simulink model "ansiOct"  (R2018a)
settings: Solver=VariableStepAuto  StartTime=0.0  StopTime=0.1  RelTol=1e-3
undefined symbols (not defined in the file or in its folder): fdesignblkfcn, G1, G2, G3, G4, G5, G6, G7, G8, gcbh, get, T
libraries: dspsrcs4 x1, dspxfrm3 x1, dspobslib x1
(part 4 of 4)

== system ansiOct/Filter Bank /Filter 6/Bandpass Filter ==
  In : Inport
  Generated Filter Block : DiscreteFir  Tag=BlockMethodSubSystem  Coefficients=[0.000758106461061279686 0.000627954496571694475 0.00074989911857348073 0.000761114809614927418 0.00061645537017629968 0.00029055864761732853 -0.000212297435837907503 -0.000851439752729806387 -0.0015505444146164738 -0.00220433141713660078 -0.00269345811208385666 -0.0029036831518041142 -0.00274902169591738832 -0.00219151013165677123 -0.00125531624779321089 -2.94406917582938247e-05 0.00133939450999522838 0.00266633068469441853 0.00375665426527416364 0.00444094125282412829 0.00460467491617639734 0.00421151448295017678 0.00331442670741950718 0.00205280067095167272 0.000623360992074421848 -0.000746056077120818887 -0.00184467664199777022 -0.00251634090714813932 -0.00269051180854619834 -0.00239906027126519364 -0.00176917093566076157 -0.000999794733265400902 -0.000319133659723472502 6.32394475281730032e-05 5.01321071435424213e-06 -0.000533853050548906464 -0.00147479661799576633 -0.00263069823207768682 -0.00373855428312695748 -0.00451152633318636226 -0.00469934145130390495 -0.00414603137021251136 -0.00282993621151281759 -0.000879477581335921387 0.00144189750548707183 0.00377984636730820025 0.00575576854269040702 0.0070395783813761879 0.00742017516255925966 0.00685102005799885071 0.00546560943815534248 0.00355583914913257899 0.00151461908209649457 -0.000243879484933040135 -0.0013739380626937134 -0.00167581523893017142 -0.0011465717235904214 1.03230104485280165e-05 0.00141982162887088629 0.00261100087096295414 0.00311849387205493864 0.00259016359212781979 0.000878201662134997008 -0.00190754912419545202 -0.00539819228084834502 -0.00901957053266398863 -0.0120944968781058152 -0.0139748575117514713 -0.0141773780990653887 -0.0124947455455883764 -0.00905835176147654596 -0.00433343430827599994 0.000953764914796475616 0.00594797445670521528 0.00983213744406967113 0.0119958323473827056 0.0121719768396738037 0.0105082726207020756 0.00755622645863471883 0.00417260028591164532 0.00134838882551079997 -4.95519307334388455e-06 0.000729964801593613257 0.00370537176846359164 0.00851975584976135368 0.0142379004449911563 0.0195242250616866828 0.0228731976908594925 0.0228998572246634224 0.0186383034187792666 0.00979080444596726156 -0.00312413315999750599 -0.0187612364695887816 -0.0350899112909813932 -0.0496717449462797875 -0.0600359549098701747 -0.0640914791889287405 -0.0605054866895300622 -0.0489815691153135183 -0.0303822329570170926 -0.00666911966071901969 0.0193385281739333406 0.044353123046185064 0.065096216944929855 0.0787880403446684502 0.0835696687708649688 0.0787880403446684502 0.065096216944929855 0.044353123046185064 0.0193385281739333406 -0.00666911966071901969 -0.0303822329570170926 -0.0489815691153135183 -0.0605054866895300622 -0.0640914791889287405 -0.0600359549098701747 -0.0496717449462797875 -0.0350899112909813932 -0.0187612364695887816 -0.00312413315999750599 0.00979080444596726156 0.0186383034187792666 0.0228998572246634224 0.0228731976908594925 0.0195242250616866828 0.0142379004449911563 0.00851975584976135368 0.00370537176846359164 0.000729964801593613257 -4.95519307334388455e-06 0.00134838882551079997 0.00417260028591164532 0.00755622645863471883 0.0105082726207020756 0.0121719768396738037 0.0119958323473827056 0.00983213744406967113 0.00594797445670521528 0.000953764914796475616 -0.00433343430827599994 -0.00905835176147654596 -0.0124947455455883764 -0.0141773780990653887 -0.0139748575117514713 -0.0120944968781058152 -0.00901957053266398863 -0.00539819228084834502 -0.00190754912419545202 0.000878201662134997008 0.00259016359212781979 0.00311849387205493864 0.00261100087096295414 0.00141982162887088629 1.03230104485280165e-05 -0.0011465717235904214 -0.00167581523893017142 -0.0013739380626937134 -0.000243879484933040135 0.00151461908209649457 0.00355583914913257899 0.00546560943815534248 0.00685102005799885071 0.00742017516255925966 0.0070395783813761879 0.00575576854269040702 0.00377984636730820025 0.00144189750548707183 -0.000879477581335921387 -0.00282993621151281759 -0.00414603137021251136 -0.00469934145130390495 ...(+954 chars)]  InputProcessing=Columns as channels (frame based)
  Out : Outport
  wires:
  In/1 -> Generated Filter Block/1
  Generated Filter Block/1 -> Out/1

== system ansiOct/Filter Bank /Filter 7/Bandpass Filter ==
  In : Inport
  Generated Filter Block : DiscreteFir  Tag=BlockMethodSubSystem  Coefficients=[2.13414128321384538e-05 -0.000759798809592844267 -0.000538552863608695817 -0.000335928687084771009 5.24523765460956263e-05 0.000389021891316683683 0.000441670017314044585 0.000201002804152968889 -5.66482041104310956e-05 4.82540718653125586e-05 0.000661195157130662703 0.00145290535972860606 0.00171570551834987831 0.000821156208601171353 -0.00122706016173827 -0.0035592211861228476 -0.0047917115473068532 -0.00384599928750740299 -0.000741273507572761032 0.0032063213974827965 0.0060143520159744784 0.00617811720942743232 0.00361378714009275709 -0.000247500764715285614 -0.00332979996628475538 -0.00420446280041711796 -0.00294244853800646518 -0.000941078759061417702 0.00015372023725453374 -0.000339198438868009507 -0.00166646070263494028 -0.00226459734106242323 -0.00102316709893813195 0.00176043503906293157 0.00447934935206520477 0.00533747013027042593 0.00367856911182492001 0.000516470990948552267 -0.00216932247011915628 -0.00287883094898484836 -0.00169248058499020288 -0.000167467028267242226 -6.72987780668683993e-05 -0.00187823875563339175 -0.00428168459721684456 -0.00506690846861694751 -0.00285578721686015379 0.00166760790483278139 0.006029145695459588 0.00763259102967875792 0.00563212788747415039 0.00158103914889088358 -0.00170186722019029756 -0.00225262242412622342 -0.000456793611400783234 0.00126212729282916547 0.000421245295943761735 -0.00337300991593043669 -0.00781216003248275462 -0.00941485970635886314 -0.00616381948463072191 0.000749146890913825582 0.00749358934481191789 0.0102174781670976728 0.00781712534353471052 0.00274298884511700114 -0.000881222608155735271 -0.00048581682164086724 0.00283594932168540004 0.00507941072064182521 0.00252652037842562068 -0.0049869822571458047 -0.0133539805431615883 -0.0168302297281559474 -0.0122504677000972589 -0.00166522433236061113 0.00877331031127788485 0.0130965766741799813 0.00988147802527619863 0.00331859676915931831 -5.62927047641235682e-05 0.00332005375214959901 0.0107486350615893823 0.0148271195132432601 0.00908621093990501227 -0.00636853670401128606 -0.0237062250686521439 -0.0321452646723445756 -0.0256095609460032132 -0.00765283884340418798 0.0104319996355094879 0.0175641674327155321 0.0113592204776215375 0.000593465033488366754 -0.00101659872684704941 0.0140099846024783047 0.0388410264823386975 0.0541897181122608512 0.0404459827764733562 -0.0071691903631041845 -0.0709724297146278466 -0.117407483937210955 -0.115558630892499958 -0.056897754248701117 0.0363871279341115711 0.120881047582533388 0.154761816480291053 0.120881047582533388 0.0363871279341115711 -0.056897754248701117 -0.115558630892499958 -0.117407483937210955 -0.0709724297146278466 -0.0071691903631041845 0.0404459827764733562 0.0541897181122608512 0.0388410264823386975 0.0140099846024783047 -0.00101659872684704941 0.000593465033488366754 0.0113592204776215375 0.0175641674327155321 0.0104319996355094879 -0.00765283884340418798 -0.0256095609460032132 -0.0321452646723445756 -0.0237062250686521439 -0.00636853670401128606 0.00908621093990501227 0.0148271195132432601 0.0107486350615893823 0.00332005375214959901 -5.62927047641235682e-05 0.00331859676915931831 0.00988147802527619863 0.0130965766741799813 0.00877331031127788485 -0.00166522433236061113 -0.0122504677000972589 -0.0168302297281559474 -0.0133539805431615883 -0.0049869822571458047 0.00252652037842562068 0.00507941072064182521 0.00283594932168540004 -0.00048581682164086724 -0.000881222608155735271 0.00274298884511700114 0.00781712534353471052 0.0102174781670976728 0.00749358934481191789 0.000749146890913825582 -0.00616381948463072191 -0.00941485970635886314 -0.00781216003248275462 -0.00337300991593043669 0.000421245295943761735 0.00126212729282916547 -0.000456793611400783234 -0.00225262242412622342 -0.00170186722019029756 0.00158103914889088358 0.00563212788747415039 0.00763259102967875792 0.006029145695459588 0.00166760790483278139 -0.00285578721686015379 -0.00506690846861694751 -0.00428168459721684456 -0.00187823875563339175 -6.72987780668683993e-05 ...(+999 chars)]  InputProcessing=Columns as channels (frame based)
  Out : Outport
  wires:
  In/1 -> Generated Filter Block/1
  Generated Filter Block/1 -> Out/1

== system ansiOct/Filter Bank /Filter 8/Bandpass Filter ==
  In : Inport
  Generated Filter Block : DiscreteFir  Tag=BlockMethodSubSystem  Coefficients=[0.00205178042206715858 -0.00532547961820776551 -0.00397094889859597993 0.012195358031550068 0.00222122035666617737 -0.0101675311674989284 -0.00207765743935300722 0.00171322319666584186 0.00316096156875898511 0.00215427953653152954 0.00151587168486719466 -0.00308404045992475076 -0.00384214539002191834 0.0018851744885105509 -0.00253203483559884387 0.00437336607375676898 0.00294255534969869613 -0.00343645491120205893 0.00315328588004639126 -0.0058993506295327066 -0.000785884496957623638 0.00289338249655475468 -0.00213829497278020557 0.00634047786545530959 -0.00142346200319672426 -0.00130023559702767888 -0.000547840818218688834 -0.00469342175639463413 0.00216874381805626367 0.000465943897917576522 0.00345059050473333316 0.0014425535928047524 -0.000948982593450888273 -0.00183374998452440511 -0.00447402606148295662 0.0014960393357583996 -0.000937944517395134241 0.00508299171121152568 0.00255221835523715629 -0.00216929628949792935 0.00114702832448088272 -0.00794272920841252936 0.00114480559439270827 0.000421889508555654781 0.00172424566773987263 0.00777065196877040499 -0.0037803304284874592 0.00149025751390483821 -0.00648412855548279564 -0.00389167514473043883 0.00316048138158256083 -0.00045542632559541753 0.00969115514074352265 -0.00133938501673315307 -1.98992606190208986e-05 -0.00462143118985150047 -0.00819999031629783763 0.00401840052744281261 -0.00198060235060348866 0.0111268243677119499 0.00219394282296035952 -0.00207355940285410033 -0.000992836248209780182 -0.0140768063677470141 0.00419075585230242135 -0.00221897275876469695 0.0092114967969341207 0.0100717321505706253 -0.00584397195126328591 0.00315636959865611168 -0.017841057873263854 -0.00083068050377322223 0.00129121433127309115 0.00390443939710146282 0.0198104690644951946 -0.00695424324712464945 0.00464326200298077144 -0.0178018047314395314 -0.0115286411909392827 0.00656786446977389218 -0.00302170447783462782 0.0303293460614103665 -0.0029211897950795554 0.00245122283332809606 -0.0127204618493201305 -0.0309732201264330716 0.0128083317281885677 -0.0106949584609893743 0.0406307977354764399 0.0143487032260006062 -0.00734434980079073148 0.00071503452988867951 -0.0694375459050317057 0.0145286523144239864 -0.016291022908200354 0.0537962623580632293 0.0844495003572756225 -0.0418618538344108365 0.0495735479967718204 -0.298100193607722941 -0.0768013077992523441 0.553042487356242063 -0.0768013077992523441 -0.298100193607722941 0.0495735479967718204 -0.0418618538344108365 0.0844495003572756225 0.0537962623580632293 -0.016291022908200354 0.0145286523144239864 -0.0694375459050317057 0.00071503452988867951 -0.00734434980079073148 0.0143487032260006062 0.0406307977354764399 -0.0106949584609893743 0.0128083317281885677 -0.0309732201264330716 -0.0127204618493201305 0.00245122283332809606 -0.0029211897950795554 0.0303293460614103665 -0.00302170447783462782 0.00656786446977389218 -0.0115286411909392827 -0.0178018047314395314 0.00464326200298077144 -0.00695424324712464945 0.0198104690644951946 0.00390443939710146282 0.00129121433127309115 -0.00083068050377322223 -0.017841057873263854 0.00315636959865611168 -0.00584397195126328591 0.0100717321505706253 0.0092114967969341207 -0.00221897275876469695 0.00419075585230242135 -0.0140768063677470141 -0.000992836248209780182 -0.00207355940285410033 0.00219394282296035952 0.0111268243677119499 -0.00198060235060348866 0.00401840052744281261 -0.00819999031629783763 -0.00462143118985150047 -1.98992606190208986e-05 -0.00133938501673315307 0.00969115514074352265 -0.00045542632559541753 0.00316048138158256083 -0.00389167514473043883 -0.00648412855548279564 0.00149025751390483821 -0.0037803304284874592 0.00777065196877040499 0.00172424566773987263 0.000421889508555654781 0.00114480559439270827 -0.00794272920841252936 0.00114702832448088272 -0.00216929628949792935 0.00255221835523715629 0.00508299171121152568 -0.000937944517395134241 0.0014960393357583996 -0.00447402606148295662 -0.00183374998452440511 -0.000948982593450888273 0.0014425535928047524 ...(+726 chars)]  InputProcessing=Columns as channels (frame based)
  Out : Outport
  wires:
  In/1 -> Generated Filter Block/1
  Generated Filter Block/1 -> Out/1
